simulink model "GNC_integrated_v3"  (R2023a)
settings: Solver=ode4  StartTime=0.0  StopTime=200  FixedStep=0.001  RelTol=1e-3
values from neighbouring files (symbols this model uses):
  baseMission = 1    [uavPackageDeliveryDataDict.sldd]
undefined symbols (not defined in the file or in its folder): Discrete, param, Time
libraries: dspfdesign x14, simulink_extras x6, uavalgslib x4, simulink x2, sharedTrackingLibrary x1, ctrlSharedLib x1, dspmtrx3 x1, SignalEditorBlockLib x1
settings Model: Creator=timme  LastModifiedBy=jipva

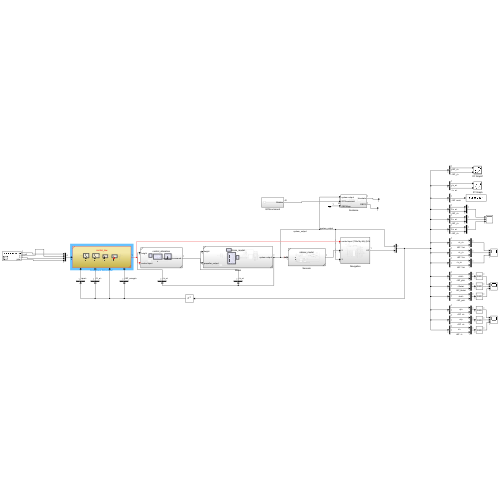
[thumbnail: Simulink's stored preview of the top-level diagram]
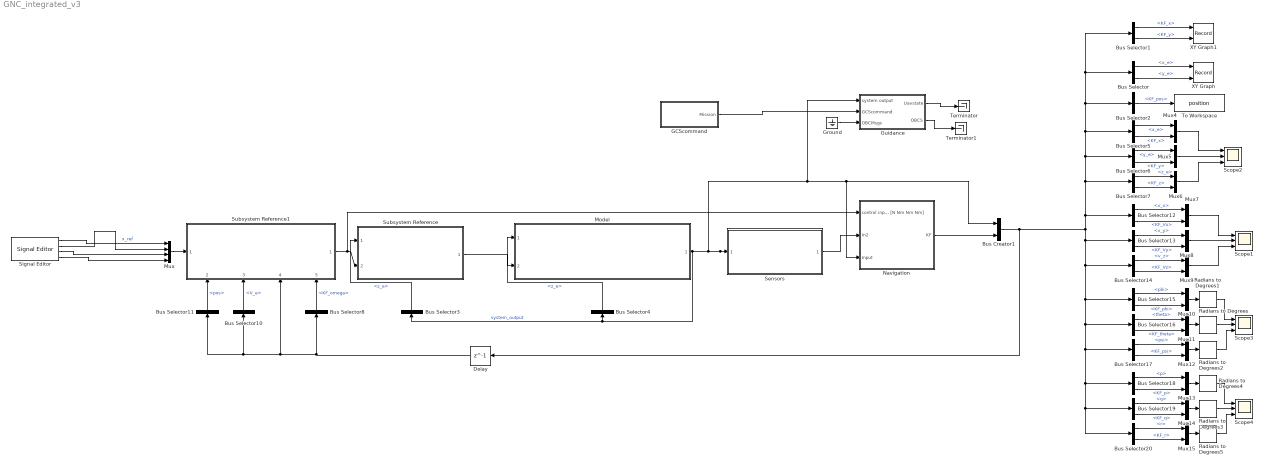
== system GNC_integrated_v3 ==
  Bus Creator1 : BusCreator  Inputs=2
  Bus Selector : BusSelector  OutputSignals=system_output.pos.x_e,system_output.pos.y_e
  Bus Selector1 : BusSelector  OutputSignals=KF.KF_pos.KF_x,KF.KF_pos.KF_y
  Bus Selector10 : BusSelector  OutputSignals=system_output.V_e
  Bus Selector11 : BusSelector  OutputSignals=system_output.pos
  Bus Selector12 : BusSelector  OutputSignals=system_output.V_e.v_x,KF.KF_vel.KF_Vx
  Bus Selector13 : BusSelector  OutputSignals=system_output.V_e.v_y,KF.KF_vel.KF_Vy
  Bus Selector14 : BusSelector  OutputSignals=system_output.V_e.v_z,KF.KF_vel.KF_Vz
  Bus Selector15 : BusSelector  OutputSignals=system_output.Att.phi,KF.KF_att.KF_phi
  Bus Selector16 : BusSelector  OutputSignals=system_output.Att.theta,KF.KF_att.KF_theta
  Bus Selector17 : BusSelector  OutputSignals=system_output.Att.psi,KF.KF_att.KF_psi
  Bus Selector18 : BusSelector  OutputSignals=system_output.ang_vel.p,KF.KF_omega.KF_p
  Bus Selector19 : BusSelector  OutputSignals=system_output.ang_vel.q,KF.KF_omega.KF_q
  Bus Selector2 : BusSelector  OutputSignals=KF.KF_pos
  Bus Selector20 : BusSelector  OutputSignals=system_output.ang_vel.r,KF.KF_omega.KF_r
  Bus Selector3 : BusSelector  OutputSignals=pos.z_e
  Bus Selector4 : BusSelector  OutputSignals=pos.z_e
  Bus Selector5 : BusSelector  OutputSignals=system_output.pos.x_e,KF.KF_pos.KF_x
  Bus Selector6 : BusSelector  OutputSignals=system_output.pos.y_e,KF.KF_pos.KF_y
  Bus Selector7 : BusSelector  OutputSignals=system_output.pos.z_e,KF.KF_pos.KF_z
  Bus Selector8 : BusSelector  OutputSignals=KF.KF_omega
  Delay : Delay  DelayLength=1
  GCScommand : Subsystem
  Ground : Ground
  Guidance : Subsystem
  Model : Subsystem  ReferencedSubsystem=drone_model
  Mux : Mux
  Mux{4..15} (12 alike) : Mux  Inputs=2
  Navigation : Subsystem
  Radians to Degrees{,1..5} (6 alike) : simulink_extras/Transformations/Radians to Degrees
  Scope{1..4} (4 alike) : Scope  NumInputPorts=3
  Sensors : Subsystem  ReferencedSubsystem=sensor_model
  Signal Editor : SignalEditorBlockLib/Signal Editor  FileName=full_system_reference.mat  ActiveScenario=StandardScenario  ActiveSignal=yaw  IsBus=off  OutputBusObjectStr=Bus: BusObject  SampleTime=param.dt  ZeroCross=off  OutputAfterFinalValue=Setting to zero  Unit=inherit  PreserveSignalName=on  ApplySigPropsToAllScenarios=on
  Subsystem Reference : Subsystem  ReferencedSubsystem=control_allocation
  Subsystem Reference1 : Subsystem  ReferencedSubsystem=control_law
      settings: PortSchema="{\"entries\":[{\"content\":{\"sides\":[{\"content\":{\"connectorIds\":[\"In1\"]},\"type\":\"ConnectorPlacement.EquallySpacedRectSide\",\"uuid\":\"cbb659e7-d19a-4e68-9ae7-e5e39426296b\"},{\"content\":{\"connectorIds\":[\"Out1\"],\"side\":\"RIGHT\"},\"type\":\"ConnectorPlacement.EquallySpacedRectSide\",\"uuid\":\"c9f08a4e-80d9-41bf-93e6-4cfd11b32426\"},{\"content\":{\"side\":\"TOP\"},\"type\":\"ConnectorPlacement.EquallySpacedRectSide\",\"uuid\":\"8eafc22d-128e-4ca7-9eba-2c3fd299252c\"},{\"content\":{\"connectorIds\":[\"In2\",\"In3\",\"In4\",\"In5\"],\"side\":\"BOTTOM\"},\"type\":\"ConnectorPlacement.EquallySpacedRectSide\",\"uuid\":\"abe1dc09-e6b8-433e-beaf-ba54ebcb4b47\"}]},\"type\":\"ConnectorPlacement.EquallySpacedConnector\",\"uuid\":\"085ffc95-65e8-4235-be8d-72c324b16b8b\"}],\"packageUris\":[\"http://schema.mathworks.com/mf0/Connector/R2020b\"],\"version\":\"1.0\"}"
  Terminator : Terminator
  Terminator1 : Terminator
  To Workspace : ToWorkspace  VariableName=position  SaveFormat=Timeseries  SampleTime=0.001
  XY Graph : Record  FileSettingsInternal="{\"entries\":[{\"content\":{\"excelSettings\":{\"content\":{},\"type\":\"Streamout.ExcelSettings\"}},\"type\":\"Streamout.FileSettingStorage\",\"uuid\":\"\"}],\"packageUris\":[\"http:\\/\\/schema.mathworks.com\\/mf0\\/streamout_blocks\\/R2020a\"],\"version\":\"1.0\"}"  Layout=[1 1]  SignalsInternal="{\"entries\":[{\"content\":{\"signals\":[{\"content\":{\"blockPath\":[],\"dimensions\":[1],\"domain\":\"\",\"lineColor\":\"#a2142f\",\"plots\":[1],\"port\":1,\"signalID\":16,\"signalName\":\"<x_e>\"},\"type\":\"RecordBlkView.Signal\",\"uuid\":\"\"},{\"content\":{\"blockPath\":[],\"dimensions\":[1],\"domain\":\"\",\"lineColor\":\"#139fff\",\"plots\":[1],\"port\":2,\"signalID\":19,\"signalName\":\"<y_e>\"},\"type\":\"RecordBlkView.Signal\",\"uuid\":\"\"}]},\"type\":\"RecordBlkView.InputSignals\",\"uuid\":\"\"}],\"packageUris\":[\"http:\\/\\/schema.mathworks.com\\/mf0\\/streamout_blocks\\/R2020a\"],\"version\":\"1.0\"}"  VisualizationBindings="{\"xyplotplugin\":{\"info\":[{\"series\":[{\"bindingParametersList\":[{\"parameter\":\"X-Axis\",\"signalID\":16,\"signalName\":\"<x_e>\"},{\"parameter\":\"Y-Axis\",\"signalID\":19,\"signalName\":\"<y_e>\"}],\"seriesID\":45778}],\"subplotID\":1}]}}"  CompatibilityTag=XY
  XY Graph1 : Record  FileSettingsInternal="{\"entries\":[{\"content\":{\"excelSettings\":{\"content\":{},\"type\":\"Streamout.ExcelSettings\"}},\"type\":\"Streamout.FileSettingStorage\",\"uuid\":\"\"}],\"packageUris\":[\"http:\\/\\/schema.mathworks.com\\/mf0\\/streamout_blocks\\/R2020a\"],\"version\":\"1.0\"}"  Layout=[1 1]  SignalsInternal="{\"entries\":[{\"content\":{\"signals\":[{\"content\":{\"blockPath\":[],\"dimensions\":[1,1],\"domain\":\"\",\"lineColor\":\"#a2142f\",\"plots\":[1],\"port\":1,\"signalID\":8,\"signalName\":\"<KF_x>\"},\"type\":\"RecordBlkView.Signal\",\"uuid\":\"\"},{\"content\":{\"blockPath\":[],\"dimensions\":[1,1],\"domain\":\"\",\"lineColor\":\"#139fff\",\"plots\":[1],\"port\":2,\"signalID\":11,\"signalName\":\"<KF_y>\"},\"type\":\"RecordBlkView.Signal\",\"uuid\":\"\"}]},\"type\":\"RecordBlkView.InputSignals\",\"uuid\":\"\"}],\"packageUris\":[\"http:\\/\\/schema.mathworks.com\\/mf0\\/streamout_blocks\\/R2020a\"],\"version\":\"1.0\"}"  VisualizationBindings="{\"xyplotplugin\":{\"info\":[{\"series\":[{\"bindingParametersList\":[{\"parameter\":\"X-Axis\",\"signalID\":8,\"signalName\":\"<KF_x>\"},{\"parameter\":\"Y-Axis\",\"signalID\":11,\"signalName\":\"<KF_y>\"}],\"seriesID\":47810}],\"subplotID\":1}]}}"  CompatibilityTag=XY
  wires:
  Bus Selector5/1 -> Mux4/1  "<x_e>"
  Bus Selector5/2 -> Mux4/2  "<KF_x>"
  Bus Selector6/1 -> Mux5/1  "<y_e>"
  Bus Selector6/2 -> Mux5/2  "<KF_y>"
  Bus Selector7/2 -> Mux6/2  "<KF_z>"
  Bus Selector7/1 -> Mux6/1  "<z_e>"
  Bus Selector12/2 -> Mux7/2  "<KF_Vx>"
  Bus Selector12/1 -> Mux7/1  "<v_x>"
  Bus Selector13/1 -> Mux8/1  "<v_y>"
  Bus Selector14/2 -> Mux9/2  "<KF_Vz>"
  Bus Selector14/1 -> Mux9/1  "<v_z>"
  Bus Selector13/2 -> Mux8/2  "<KF_Vy>"
  Bus Selector16/2 -> Mux11/2  "<KF_theta>"
  Mux12/1 -> Radians to Degrees2/1
  Mux11/1 -> Radians to Degrees/1
  Bus Selector17/2 -> Mux12/2  "<KF_psi>"
  Bus Selector17/1 -> Mux12/1  "<psi>"
  Bus Selector15/2 -> Mux10/2  "<KF_phi>"
  Mux10/1 -> Radians to Degrees1/1
  Bus Selector15/1 -> Mux10/1  "<phi>"
  Bus Selector16/1 -> Mux11/1  "<theta>"
  Bus Selector19/2 -> Mux14/2  "<KF_q>"
  Bus Selector18/2 -> Mux13/2  "<KF_p>"
  Mux13/1 -> Radians to Degrees4/1
  Bus Selector20/1 -> Mux15/1  "<r>"
  Bus Selector18/1 -> Mux13/1  "<p>"
  Mux15/1 -> Radians to Degrees5/1
  Bus Selector20/2 -> Mux15/2  "<KF_r>"
  Mux14/1 -> Radians to Degrees3/1
  Bus Selector19/1 -> Mux14/1  "<q>"
  Signal Editor/1 -> Mux/1  "x_ref"
  Bus Selector/1 -> XY Graph/1  "<x_e>"
  Bus Selector/2 -> XY Graph/2  "<y_e>"
  Mux5/1 -> Scope2/2
  Mux4/1 -> Scope2/1
  Mux6/1 -> Scope2/3
  Mux8/1 -> Scope1/2
  Mux9/1 -> Scope1/3
  Mux7/1 -> Scope1/1
  Radians to Degrees2/1 -> Scope3/3
  Radians to Degrees1/1 -> Scope3/1
  Radians to Degrees/1 -> Scope3/2
  Radians to Degrees5/1 -> Scope4/3
  Radians to Degrees4/1 -> Scope4/1
  Radians to Degrees3/1 -> Scope4/2
  Bus Selector1/1 -> XY Graph1/1  "<KF_x>"
  Bus Selector1/2 -> XY Graph1/2  "<KF_y>"
  Sensors/1 -> Navigation/2(In2)
  Navigation/1(KF) -> Bus Creator1/2
  Bus Selector2/1 -> To Workspace/1  "<KF_pos>"
  Bus Creator1/1 -> Delay/1, Bus Selector13/1, Bus Selector14/1, Bus Selector20/1, Bus Selector19/1, Bus Selector18/1, Bus Selector17/1, Bus Selector16/1, Bus Selector15/1, Bus Selector12/1, Bus Selector7/1, Bus Selector6/1, Bus Selector2/1, Bus Selector1/1, Bus Selector/1, Bus Selector5/1
  Mux/1 -> Subsystem Reference1/1
  Bus Selector11/1 -> Subsystem Reference1/2  "<pos>"
  Bus Selector10/1 -> Subsystem Reference1/3  "<V_e>"
  Delay/1 -> Bus Selector8/1, Subsystem Reference1/4, Bus Selector11/1, Bus Selector10/1
  Bus Selector8/1 -> Subsystem Reference1/5  "<KF_omega>"
  Bus Selector3/1 -> Subsystem Reference/1  "<z_e>"
  Bus Selector4/1 -> Model/1  "<z_e>"
  Signal Editor/4 -> Mux/4
  Signal Editor/3 -> Mux/3
  Signal Editor/2 -> Mux/2
  Subsystem Reference1/1 -> Subsystem Reference/2, Navigation/1(control input (T Mx My Mz) [N Nm Nm Nm])
  Subsystem Reference/1 -> Model/2
  Model/1 -> Bus Selector3/1, Bus Selector4/1, Sensors/1, Guidance/1(system output), Navigation/3(Input), Bus Creator1/1  "system_output"
  Guidance/2(OBCS) -> Terminator1/1
  Ground/1 -> Guidance/3(OBCMsgs)
  Guidance/1(Uavstate) -> Terminator/1
  GCScommand/1(Mission) -> Guidance/2(GCScommand)

== system GNC_integrated_v3/GCScommand ==
  Constant : Constant  Value=baseMission  OutDataTypeStr=Bus: UAVPathManagerBus  SampleTime=-1
  Mission : Outport
  wires:
  Constant/1 -> Mission/1

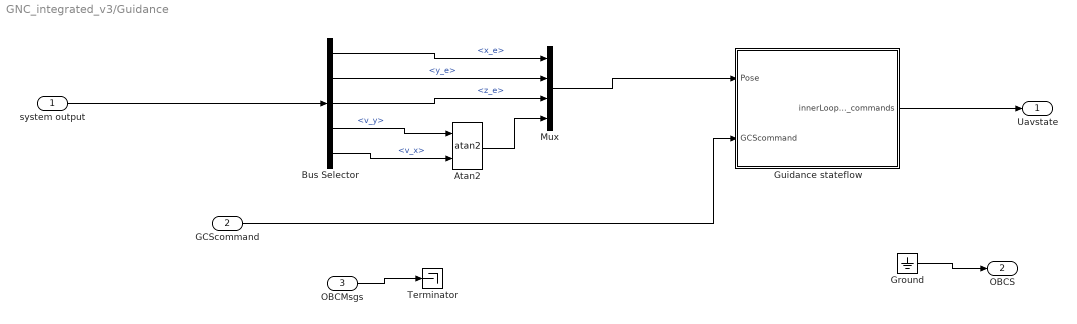
== system GNC_integrated_v3/Guidance ==
  system output : Inport
  GCScommand : Inport  Port=2
  OBCMsgs : Inport  Port=3
  Atan2 : Trigonometry  Operator=atan2
  Bus Selector : BusSelector  OutputSignals=pos.x_e,pos.y_e,pos.z_e,V_e.v_y,V_e.v_x
  Ground : Ground
  Guidance stateflow : Subsystem
  Mux : Mux
  Terminator : Terminator
  Uavstate : Outport
  OBCS : Outport  Port=2
  wires:
  Bus Selector/4 -> Atan2/1  "<v_y>"
  Bus Selector/5 -> Atan2/2  "<v_x>"
  Bus Selector/3 -> Mux/3  "<z_e>"
  Bus Selector/2 -> Mux/2  "<y_e>"
  Bus Selector/1 -> Mux/1  "<x_e>"
  Atan2/1 -> Mux/4
  Mux/1 -> Guidance stateflow/1(Pose)
  GCScommand/1 -> Guidance stateflow/2(GCScommand)
  OBCMsgs/1 -> Terminator/1
  Guidance stateflow/1(innerLoop_commands) -> Uavstate/1
  Ground/1 -> OBCS/1
  system output/1 -> Bus Selector/1

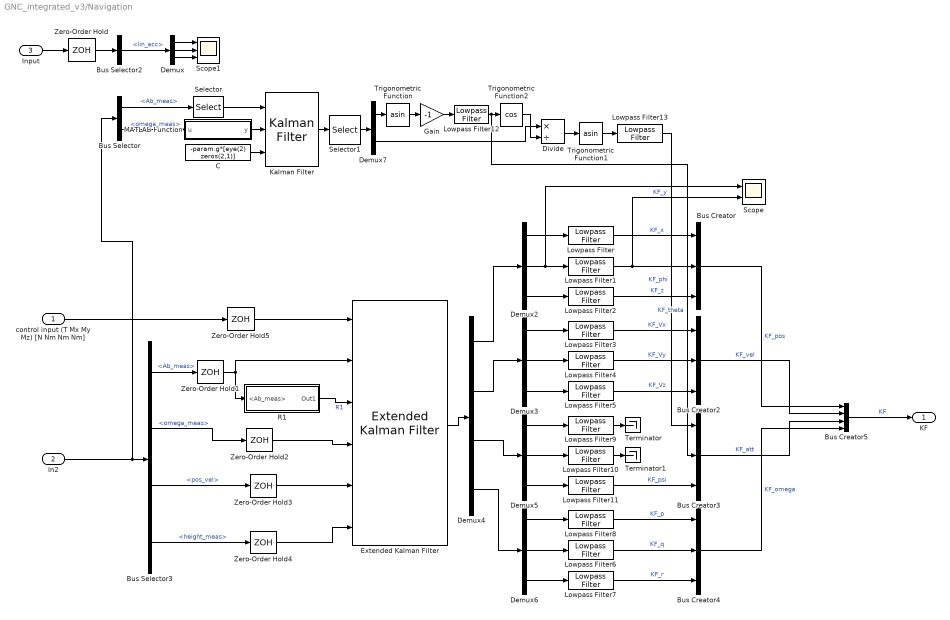
== system GNC_integrated_v3/Navigation ==
  control input (T Mx My Mz) [N Nm Nm Nm] : Inport
  In2 : Inport  Port=2
  Input : Inport  Port=3
  Bus Creator{,2..4} (4 alike) : BusCreator  Inputs=3
  Bus Creator5 : BusCreator  Inputs=4
  Bus Selector : BusSelector  OutputSignals=Ab_meas,omega_meas
  Bus Selector2 : BusSelector  OutputSignals=lin_acc
  Bus Selector3 : BusSelector  OutputSignals=Ab_meas,omega_meas,pos_vel,height_meas
  C : Constant  Value=-param.g*[eye(2) zeros(2,1)]
  Demux{,2..3,5..6} (5 alike) : Demux  Outputs=3
  Demux4 : Demux
  Demux7 : Demux  Outputs=2
  Divide : Product  Inputs=*/
  Extended Kalman Filter : sharedTrackingLibrary/Extended Kalman Filter  StateTransitionFcn=stateTransition  HasStateTransitionJacobianFcn=off  HasAdditiveProcessNoise=Additive  ProcessNoise=diag([1*ones(1,6) [1 1 0.01] [0.1 0.1 0.1]])  HasTimeVaryingProcessNoise=off  HasStateTransitionFcnExtraArgument=1  InitialState=zeros(12,1)  InitialStateCovariance=zeros(12)  MeasurementFcn1=accelerometer_model  HasMeasurementJacobianFcn1=off  HasMeasurementEnablePort1=off  HasAdditiveMeasurementNoise1=Additive  MeasurementNoise1=diag([20 20 20])  HasTimeVaryingMeasurementNoise1=on  HasMeasurementFcnExtraArgument1=0  HasMeasurementWrapping1=off  MeasurementFcn2=gyrometer_model  HasMeasurementJacobianFcn2=off  HasMeasurementEnablePort2=off  HasAdditiveMeasurementNoise2=Additive  MeasurementNoise2=diag([1 1 10])  HasTimeVaryingMeasurementNoise2=off  HasMeasurementFcnExtraArgument2=0  HasMeasurementWrapping2=off  MeasurementFcn3=GPS_model  HasMeasurementJacobianFcn3=off  HasMeasurementEnablePort3=off  HasAdditiveMeasurementNoise3=Additive  MeasurementNoise3=diag([0.001 0.001 0.001 0.001 0.001 0.001])  HasTimeVaryingMeasurementNoise3=off  HasMeasurementFcnExtraArgument3=0  HasMeasurementWrapping3=off  MeasurementFcn4=Barometer_model  HasMeasurementJacobianFcn4=off  HasMeasurementEnablePort4=off  HasAdditiveMeasurementNoise4=Additive  MeasurementNoise4=0.01  HasTimeVaryingMeasurementNoise4=off  HasMeasurementFcnExtraArgument4=0  HasMeasurementWrapping4=off  MeasurementFcn5=myMeasurementFcn  HasMeasurementJacobianFcn5=off  HasMeasurementEnablePort5=off  HasAdditiveMeasurementNoise5=Additive  MeasurementNoise5=1  HasTimeVaryingMeasurementNoise5=off  HasMeasurementFcnExtraArgument5=0  HasMeasurementWrapping5=off  EnableMultirate=on  StateTransitionFcnSampleTime=0.001  MeasurementFcn1SampleTime=0.001  MeasurementFcn2SampleTime=0.001  MeasurementFcn3SampleTime=0.001  MeasurementFcn4SampleTime=0.01  MeasurementFcn5SampleTime=1  UseCurrentEstimator=on  OutputStateCovariance=off  DataType=double  SampleTime=0.001  NumberOfMeasurements=4
  Gain : Gain  Gain=-1
  Kalman Filter : ctrlSharedLib/Kalman Filter  TimeDomain=Discrete-Time  UseCurrentEstimator=on  ModelSource=Input port  ModelSourceVariable=ss(0.95,1,1,0,1)  A=0.95  B=1  C=1  D=0  NumberOfStates=3  NumberOfInputs=1  NumberOfOutputs=2  InitialEstimateSource=Dialog  X0=0  P0=1  UseK=off  UseGH=off  NumberOfProcessNoiseInputs=1  G=eye(3)  TimeInvariantG=on  H=ones(2,1)  TimeInvariantH=on  Q=100  TimeInvariantQ=on  R=0.0001  TimeInvariantR=on  N=0  TimeInvariantN=on  AddInputPort=off  AddEnablePort=off  OutputEstimatedY=off  OutputP=off  Ts=0.001
  Lowpass Filter : dspfdesign/Lowpass Filter  FilterType=IIR  DesignForMinimumOrder=on  FilterOrder=50  PassbandFrequency=1  StopbandFrequency=499  PassbandRipple=0.1  StopbandAttenuation=80  SampleRateMode=Specify on dialog  SampleRate=1000  SimulateUsing=Interpreted execution  roundingMode=Floor  coeffsDataTypeStr=fixdt(1,16)
  Lowpass Filter1 : dspfdesign/Lowpass Filter  FilterType=IIR  DesignForMinimumOrder=on  FilterOrder=50  PassbandFrequency=1  StopbandFrequency=499  PassbandRipple=0.1  StopbandAttenuation=80  SampleRateMode=Specify on dialog  SampleRate=1000  SimulateUsing=Interpreted execution  roundingMode=Floor  coeffsDataTypeStr=fixdt(1,16)
  Lowpass Filter10 : dspfdesign/Lowpass Filter  FilterType=IIR  DesignForMinimumOrder=on  FilterOrder=50  PassbandFrequency=0.1  StopbandFrequency=25  PassbandRipple=0.1  StopbandAttenuation=80  SampleRateMode=Specify on dialog  SampleRate=1000  SimulateUsing=Interpreted execution  roundingMode=Floor  coeffsDataTypeStr=fixdt(1,16)
  Lowpass Filter11 : dspfdesign/Lowpass Filter  FilterType=IIR  DesignForMinimumOrder=on  FilterOrder=50  PassbandFrequency=0.1  StopbandFrequency=25  PassbandRipple=0.1  StopbandAttenuation=80  SampleRateMode=Specify on dialog  SampleRate=1000  SimulateUsing=Interpreted execution  roundingMode=Floor  coeffsDataTypeStr=fixdt(1,16)
  Lowpass Filter{6..8,12..13} (5 alike) : dspfdesign/Lowpass Filter  FilterType=IIR  DesignForMinimumOrder=on  FilterOrder=50  PassbandFrequency=5  StopbandFrequency=60  PassbandRipple=0.1  StopbandAttenuation=45  SampleRateMode=Specify on dialog  SampleRate=1000  SimulateUsing=Interpreted execution  roundingMode=Floor  coeffsDataTypeStr=fixdt(1,16)
  Lowpass Filter2 : dspfdesign/Lowpass Filter  FilterType=IIR  DesignForMinimumOrder=on  FilterOrder=50  PassbandFrequency=1  StopbandFrequency=499  PassbandRipple=0.1  StopbandAttenuation=80  SampleRateMode=Specify on dialog  SampleRate=1000  SimulateUsing=Interpreted execution  roundingMode=Floor  coeffsDataTypeStr=fixdt(1,16)
  Lowpass Filter3 : dspfdesign/Lowpass Filter  FilterType=IIR  DesignForMinimumOrder=on  FilterOrder=50  PassbandFrequency=0.1  StopbandFrequency=10  PassbandRipple=0.1  StopbandAttenuation=80  SampleRateMode=Specify on dialog  SampleRate=1000  SimulateUsing=Interpreted execution  roundingMode=Floor  coeffsDataTypeStr=fixdt(1,16)
  Lowpass Filter4 : dspfdesign/Lowpass Filter  FilterType=IIR  DesignForMinimumOrder=on  FilterOrder=50  PassbandFrequency=0.1  StopbandFrequency=50  PassbandRipple=0.1  StopbandAttenuation=80  SampleRateMode=Specify on dialog  SampleRate=1000  SimulateUsing=Interpreted execution  roundingMode=Floor  coeffsDataTypeStr=fixdt(1,16)
  Lowpass Filter5 : dspfdesign/Lowpass Filter  FilterType=IIR  DesignForMinimumOrder=on  FilterOrder=50  PassbandFrequency=0.1  StopbandFrequency=50  PassbandRipple=0.1  StopbandAttenuation=80  SampleRateMode=Specify on dialog  SampleRate=1000  SimulateUsing=Interpreted execution  roundingMode=Floor  coeffsDataTypeStr=fixdt(1,16)
  Lowpass Filter9 : dspfdesign/Lowpass Filter  FilterType=IIR  DesignForMinimumOrder=on  FilterOrder=50  PassbandFrequency=0.1  StopbandFrequency=25  PassbandRipple=0.1  StopbandAttenuation=80  SampleRateMode=Specify on dialog  SampleRate=1000  SimulateUsing=Interpreted execution  roundingMode=Floor  coeffsDataTypeStr=fixdt(1,16)
  MATLAB Function : MATLAB Function  TreatAsAtomicUnit=on
  R1 : Subsystem
  Scope : Scope  NumInputPorts=2
  Scope1 : Scope  NumInputPorts=3
  Selector : Selector  InputPortWidth=3  IndexOptions=Index vector (dialog)  Indices=[1 2]  OutputSizes=1
  Selector1 : Selector  InputPortWidth=3  IndexOptions=Index vector (dialog)  Indices=[1 2]  OutputSizes=1
  Terminator : Terminator
  Terminator1 : Terminator
  Trigonometric Function : Trigonometry  Operator=asin
  Trigonometric Function1 : Trigonometry  Operator=asin
  Trigonometric Function2 : Trigonometry  Operator=cos
  Zero-Order Hold{,1..3,5} (5 alike) : ZeroOrderHold  SampleTime=0.001
  Zero-Order Hold4 : ZeroOrderHold  SampleTime=0.01
  KF : Outport
  wires:
  Demux5/2 -> Lowpass Filter10/1
  Bus Selector3/2 -> Zero-Order Hold2/1  "<omega_meas>"
  Bus Selector3/3 -> Zero-Order Hold3/1  "<pos_vel>"
  Demux2/3 -> Lowpass Filter2/1
  Zero-Order Hold5/1 -> Extended Kalman Filter/1
  Demux3/1 -> Lowpass Filter3/1
  In2/1 -> Bus Selector3/1, Bus Selector/1
  Demux5/3 -> Lowpass Filter11/1
  Bus Creator2/1 -> Bus Creator5/2  "KF_vel"
  Bus Creator/1 -> Bus Creator5/1  "KF_pos"
  Demux4/2 -> Demux3/1
  Demux3/3 -> Lowpass Filter5/1
  Demux2/1 -> Lowpass Filter/1
  Demux4/1 -> Demux2/1
  Demux5/1 -> Lowpass Filter9/1
  Zero-Order Hold1/1 -> Extended Kalman Filter/2, R1/1(<Ab_meas>)
  Demux3/2 -> Lowpass Filter4/1
  Bus Selector3/4 -> Zero-Order Hold4/1  "<height_meas>"
  Bus Creator3/1 -> Bus Creator5/3  "KF_att"
  Demux4/4 -> Demux6/1
  Lowpass Filter1/1 -> Scope/2, Bus Creator/2  "KF_y"
  Extended Kalman Filter/1 -> Demux4/1
  Demux4/3 -> Demux5/1
  Bus Creator5/1 -> KF/1  "KF"
  control input (T Mx My Mz) [N Nm Nm Nm]/1 -> Zero-Order Hold5/1
  Lowpass Filter/1 -> Bus Creator/1  "KF_x"
  Demux2/2 -> Scope/1, Lowpass Filter1/1
  Lowpass Filter2/1 -> Bus Creator/3  "KF_z"
  Lowpass Filter3/1 -> Bus Creator2/1  "KF_Vx"
  Lowpass Filter4/1 -> Bus Creator2/2  "KF_Vy"
  Lowpass Filter5/1 -> Bus Creator2/3  "KF_Vz"
  Lowpass Filter11/1 -> Bus Creator3/3  "KF_psi"
  Lowpass Filter8/1 -> Bus Creator4/1  "KF_p"
  Lowpass Filter6/1 -> Bus Creator4/2  "KF_q"
  Lowpass Filter7/1 -> Bus Creator4/3  "KF_r"
  Demux6/1 -> Lowpass Filter8/1
  Demux6/2 -> Lowpass Filter6/1
  Demux6/3 -> Lowpass Filter7/1
  Zero-Order Hold2/1 -> Extended Kalman Filter/4
  Zero-Order Hold3/1 -> Extended Kalman Filter/5
  Zero-Order Hold4/1 -> Extended Kalman Filter/6
  R1/1(Out1) -> Extended Kalman Filter/3  "R1"
  Bus Selector3/1 -> Zero-Order Hold1/1  "<Ab_meas>"
  Bus Creator4/1 -> Bus Creator5/4  "KF_omega"
  Bus Selector/1 -> Selector/1  "<Ab_meas>"
  C/1 -> Kalman Filter/3
  Bus Selector/2 -> MATLAB Function/1(u)  "<omega_meas>"
  MATLAB Function/1(y) -> Kalman Filter/2
  Kalman Filter/1 -> Selector1/1
  Demux7/1 -> Trigonometric Function/1
  Selector/1 -> Kalman Filter/1
  Gain/1 -> Lowpass Filter12/1
  Trigonometric Function/1 -> Gain/1
  Demux7/2 -> Divide/1
  Lowpass Filter12/1 -> Bus Creator3/2, Trigonometric Function2/1  "KF_theta"
  Input/1 -> Zero-Order Hold/1
  Zero-Order Hold/1 -> Bus Selector2/1
  Lowpass Filter13/1 -> Bus Creator3/1  "KF_phi"
  Divide/1 -> Trigonometric Function1/1
  Selector1/1 -> Demux7/1
  Trigonometric Function1/1 -> Lowpass Filter13/1
  Trigonometric Function2/1 -> Divide/2
  Lowpass Filter9/1 -> Terminator/1
  Lowpass Filter10/1 -> Terminator1/1
  Bus Selector2/1 -> Demux/1  "<lin_acc>"
  Demux/2 -> Scope1/2
  Demux/1 -> Scope1/1
  Demux/3 -> Scope1/3

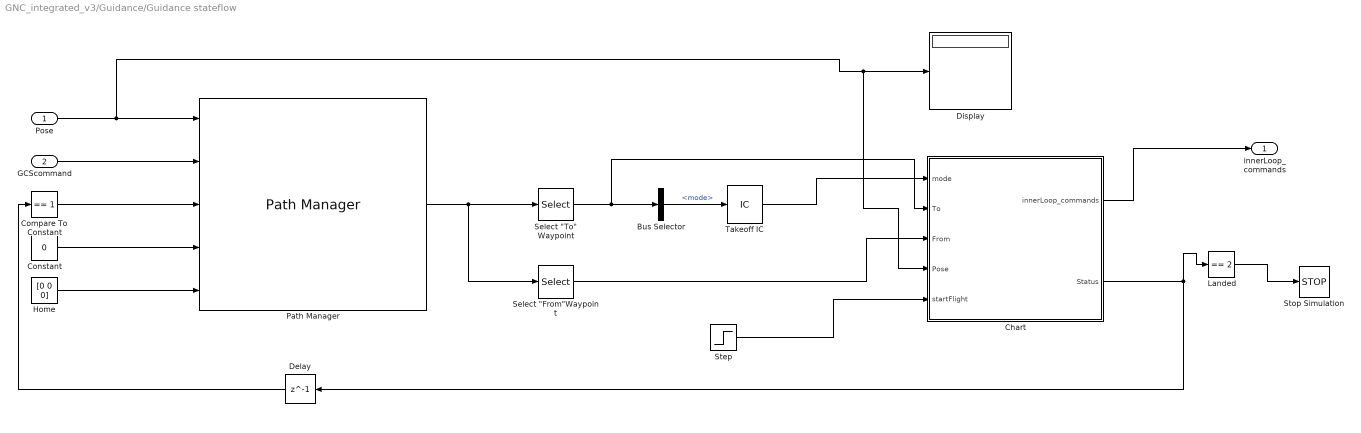
== system GNC_integrated_v3/Guidance/Guidance stateflow ==
  Pose : Inport
  GCScommand : Inport  Port=2
  Bus Selector : BusSelector  OutputSignals=mode
  Chart : Stateflow chart  TreatAsAtomicUnit=on
  Compare To Constant : simulink/Logic and Bit Operations/Compare To Constant  relop===  const=1  OutDataTypeStr=boolean
  Constant : Constant  Value=0  OutDataTypeStr=uint8
  Delay : Delay  DelayLength=1  InitialCondition=0
  Display : Display
  Home : Constant  Value=[0 0 0]
  Landed : simulink/Logic and Bit Operations/Compare To Constant  relop===  const=2  OutDataTypeStr=boolean
  Path Manager : uavalgslib/Path Manager  UAVType=multirotor  LoiterRadius=25  dataType=single  inputBusName='UAVPathManagerBus'  SimulateUsing=Code generation
  "Select \"From\"Waypoint" : Selector  InputPortWidth=2  IndexOptions=Index vector (dialog)  Indices=2  OutputSizes=1
  "Select \"To\" Waypoint" : Selector  InputPortWidth=2  IndexOptions=Index vector (dialog)  Indices=1  OutputSizes=1
  Step : Step  Time=0.5  SampleTime=0.02
  Stop Simulation : Stop
  Takeoff IC : InitialCondition
  innerLoop_commands : Outport
  wires:
  GCScommand/1 -> Path Manager/2
  Home/1 -> Path Manager/5
  Constant/1 -> Path Manager/4
  Path Manager/1 -> "Select \"From\"Waypoint"/1, "Select \"To\" Waypoint"/1
  Bus Selector/1 -> Takeoff IC/1  "<mode>"
  Delay/1 -> Compare To Constant/1
  Compare To Constant/1 -> Path Manager/3
  Step/1 -> Chart/5(startFlight)
  Landed/1 -> Stop Simulation/1
  Pose/1 -> Chart/4(Pose), Display/1, Path Manager/1
  "Select \"To\" Waypoint"/1 -> Chart/2(To), Bus Selector/1
  "Select \"From\"Waypoint"/1 -> Chart/3(From)
  Takeoff IC/1 -> Chart/1(mode)
  Chart/1(innerLoop_commands) -> innerLoop_commands/1
  Chart/2(Status) -> Landed/1, Delay/1

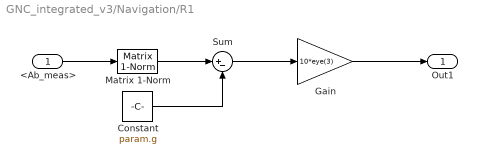
== system GNC_integrated_v3/Navigation/R1 ==
  <Ab_meas> : Inport
  Constant : Constant  Value=param.g
  Gain : Gain  Gain=10*eye(3)
  Matrix 1-Norm : dspmtrx3/Matrix  1-Norm  roundingMode=Floor  overflowMode=off  outputDataTypeStr=Inherit: Same as accumulator  outputMin=[]  outputMax=[]  outputLastDataTypeStr=Inherit: Same as accumulator
  Sum : Sum  Inputs=|+-
  Out1 : Outport
  wires:
  Matrix 1-Norm/1 -> Sum/1
  <Ab_meas>/1 -> Matrix 1-Norm/1
  Constant/1 -> Sum/2
  Sum/1 -> Gain/1
  Gain/1 -> Out1/1

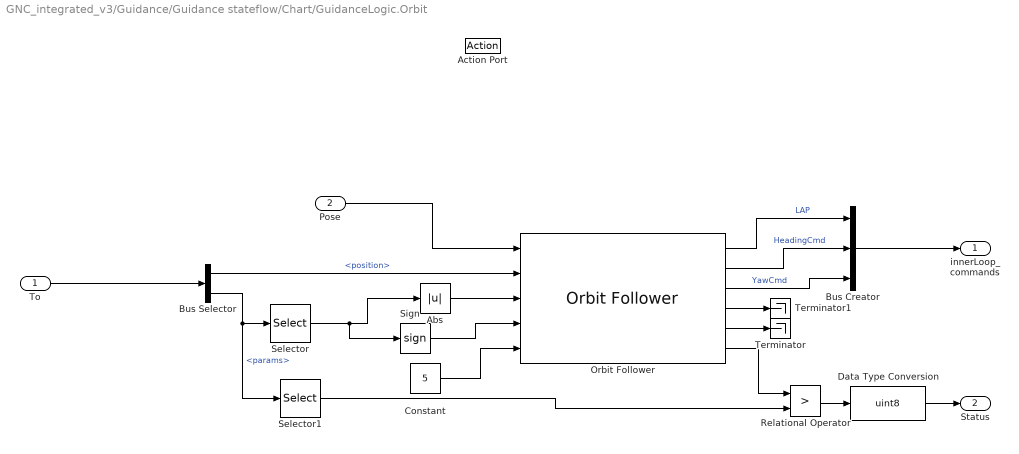
== system GNC_integrated_v3/Guidance/Guidance stateflow/Chart/GuidanceLogic.Orbit ==
  To : Inport
  Pose : Inport  Port=2
  Action Port : ActionPort
      settings: CopyFcn=Stateflow.SLINSF.SimulinkMan.removeBlockPreDeleteFcn  PreDeleteFcn=Stateflow.SLINSF.SimulinkMan.unsafePredeleteFcn
  Abs : Abs  SaturateOnIntegerOverflow=off
  Bus Creator : BusCreator  Inputs=3  OutDataTypeStr=Bus: innerLoopCmdsBus  NonVirtualBus=on
  Bus Selector : BusSelector  OutputSignals=position,params
  Constant : Constant  Value=5  OutDataTypeStr=uint8
  Data Type Conversion : DataTypeConversion  OutDataTypeStr=uint8  SaturateOnIntegerOverflow=off  RndMeth=Floor
  Orbit Follower : uavalgslib/Orbit Follower  UAVType=multirotor  MinOrbitRadius=1  MinLookaheadDistance=0.1  ExternalReset=none  ShowCrossTrackErrorOutput=off  ShowNumTurnsOutput=on  SimulateUsing=Code generation
  Relational Operator : RelationalOperator  Operator=>  OutDataTypeStr=boolean  RndMeth=Simplest  InputSameDT=off
  Selector : Selector  InputPortWidth=4  IndexOptions=Index vector (dialog)  Indices=[3]  OutputSizes=1
  Selector1 : Selector  InputPortWidth=4  IndexOptions=Index vector (dialog)  Indices=[1]  OutputSizes=1
  Sign : Signum
  Terminator : Terminator
  Terminator1 : Terminator
  innerLoop_commands : Outport
  Status : Outport  Port=2
  wires:
  To/1 -> Bus Selector/1
  Orbit Follower/4 -> Terminator1/1
  Orbit Follower/5 -> Terminator/1
  Orbit Follower/1 -> Bus Creator/1  "LAP"
  Orbit Follower/2 -> Bus Creator/2  "HeadingCmd"
  Orbit Follower/3 -> Bus Creator/3  "YawCmd"
  Bus Creator/1 -> innerLoop_commands/1
  Pose/1 -> Orbit Follower/1
  Bus Selector/1 -> Orbit Follower/2  "<position>"
  Bus Selector/2 -> Selector1/1, Selector/1  "<params>"
  Abs/1 -> Orbit Follower/3
  Selector/1 -> Sign/1, Abs/1
  Constant/1 -> Orbit Follower/5
  Sign/1 -> Orbit Follower/4
  Orbit Follower/6 -> Relational Operator/1
  Selector1/1 -> Relational Operator/2
  Relational Operator/1 -> Data Type Conversion/1
  Data Type Conversion/1 -> Status/1

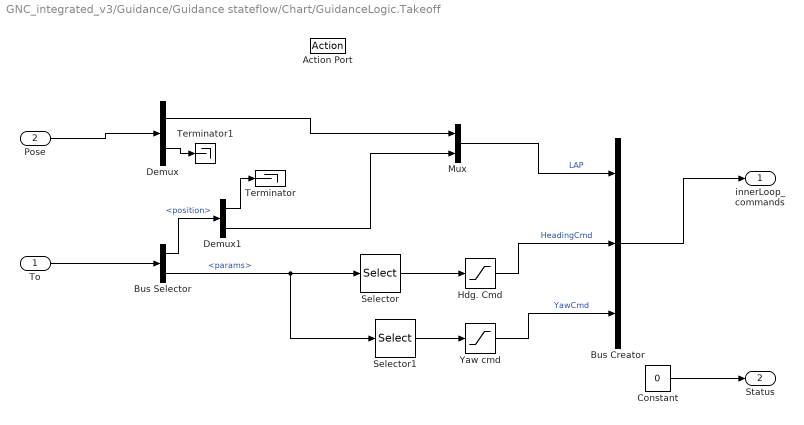
== system GNC_integrated_v3/Guidance/Guidance stateflow/Chart/GuidanceLogic.Takeoff ==
  To : Inport
  Pose : Inport  Port=2
  Action Port : ActionPort
      settings: CopyFcn=Stateflow.SLINSF.SimulinkMan.removeBlockPreDeleteFcn  PreDeleteFcn=Stateflow.SLINSF.SimulinkMan.unsafePredeleteFcn
  Bus Creator : BusCreator  Inputs=3  OutDataTypeStr=Bus: innerLoopCmdsBus  NonVirtualBus=on
  Bus Selector : BusSelector  OutputSignals=position,params
  Constant : Constant  Value=0
  Demux : Demux  Outputs=[2 2]
  Demux1 : Demux  Outputs=2
  Hdg. Cmd : Saturate
  Mux : Mux  Inputs=2
  Selector : Selector  InputPortWidth=4  IndexOptions=Index vector (dialog)  Indices=4  OutputSizes=1
  Selector1 : Selector  InputPortWidth=4  IndexOptions=Index vector (dialog)  Indices=4  OutputSizes=1
  Terminator : Terminator
  Terminator1 : Terminator
  Yaw cmd : Saturate  UpperLimit=pi  LowerLimit=-pi
  innerLoop_commands : Outport
  Status : Outport  Port=2  OutDataTypeStr=uint8
  wires:
  Pose/1 -> Demux/1
  Demux/1 -> Mux/1
  Mux/1 -> Bus Creator/1  "LAP"
  To/1 -> Bus Selector/1
  Bus Selector/1 -> Demux1/1  "<position>"
  Demux1/1 -> Terminator/1
  Demux1/2 -> Mux/2
  Bus Selector/2 -> Selector1/1, Selector/1  "<params>"
  Bus Creator/1 -> innerLoop_commands/1
  Demux/2 -> Terminator1/1
  Hdg. Cmd/1 -> Bus Creator/2  "HeadingCmd"
  Selector1/1 -> Yaw cmd/1
  Selector/1 -> Hdg. Cmd/1
  Yaw cmd/1 -> Bus Creator/3  "YawCmd"
  Constant/1 -> Status/1

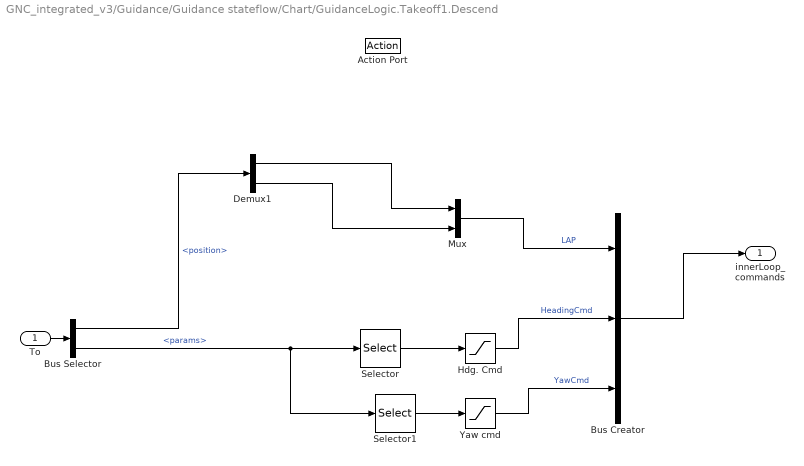
== system GNC_integrated_v3/Guidance/Guidance stateflow/Chart/GuidanceLogic.Takeoff1.Descend ==
  To : Inport
  Action Port : ActionPort
      settings: CopyFcn=Stateflow.SLINSF.SimulinkMan.removeBlockPreDeleteFcn  PreDeleteFcn=Stateflow.SLINSF.SimulinkMan.unsafePredeleteFcn
  Bus Creator : BusCreator  Inputs=3  OutDataTypeStr=Bus: innerLoopCmdsBus  NonVirtualBus=on
  Bus Selector : BusSelector  OutputSignals=position,params
  Demux1 : Demux  Outputs=[2 1]
  Hdg. Cmd : Saturate
  Mux : Mux  Inputs=2
  Selector : Selector  InputPortWidth=4  IndexOptions=Index vector (dialog)  Indices=4  OutputSizes=1
  Selector1 : Selector  InputPortWidth=4  IndexOptions=Index vector (dialog)  Indices=4  OutputSizes=1
  Yaw cmd : Saturate  UpperLimit=pi  LowerLimit=-pi
  innerLoop_commands : Outport
  wires:
  Bus Selector/1 -> Demux1/1  "<position>"
  Demux1/2 -> Mux/2
  Mux/1 -> Bus Creator/1  "LAP"
  Bus Selector/2 -> Selector1/1, Selector/1  "<params>"
  Selector1/1 -> Yaw cmd/1
  Demux1/1 -> Mux/1
  Hdg. Cmd/1 -> Bus Creator/2  "HeadingCmd"
  Selector/1 -> Hdg. Cmd/1
  Yaw cmd/1 -> Bus Creator/3  "YawCmd"
  Bus Creator/1 -> innerLoop_commands/1
  To/1 -> Bus Selector/1

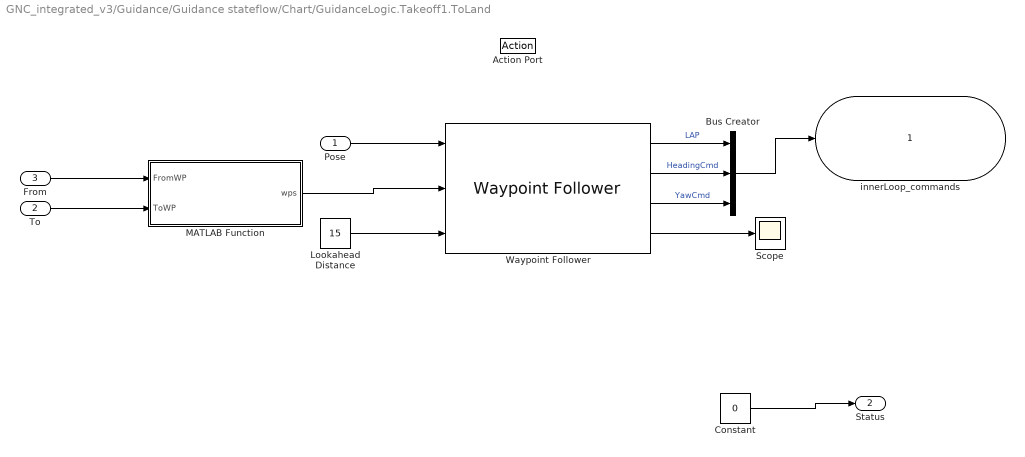
== system GNC_integrated_v3/Guidance/Guidance stateflow/Chart/GuidanceLogic.Takeoff1.ToLand ==
  Pose : Inport
  To : Inport  Port=2
  From : Inport  Port=3
  Action Port : ActionPort
      settings: CopyFcn=Stateflow.SLINSF.SimulinkMan.removeBlockPreDeleteFcn  PreDeleteFcn=Stateflow.SLINSF.SimulinkMan.unsafePredeleteFcn
  Bus Creator : BusCreator  Inputs=3  OutDataTypeStr=Bus: innerLoopCmdsBus  NonVirtualBus=on
  Constant : Constant  Value=0
  Lookahead Distance : Constant  Value=15
  MATLAB Function : MATLAB Function  TreatAsAtomicUnit=on
  Scope : Scope
  Waypoint Follower : uavalgslib/Waypoint Follower  UAVType=multirotor  StartFrom=first  TransitionRadiusSource=internal  TransitionRadius=10  MinLookaheadDistance=0.1  YawInput=off  ShowCrossTrackErrorOutput=off  ShowStatusOutput=off  SimulateUsing=Interpreted execution
  innerLoop_commands : Outport  OutDataTypeStr=Bus: innerLoopCmdsBus
  Status : Outport  Port=2
  wires:
  To/1 -> MATLAB Function/2(ToWP)
  MATLAB Function/1(wps) -> Waypoint Follower/2
  Waypoint Follower/1 -> Bus Creator/1  "LAP"
  Bus Creator/1 -> innerLoop_commands/1
  From/1 -> MATLAB Function/1(FromWP)
  Pose/1 -> Waypoint Follower/1
  Waypoint Follower/2 -> Bus Creator/2  "HeadingCmd"
  Waypoint Follower/4 -> Scope/1
  Lookahead Distance/1 -> Waypoint Follower/3
  Waypoint Follower/3 -> Bus Creator/3  "YawCmd"
  Constant/1 -> Status/1

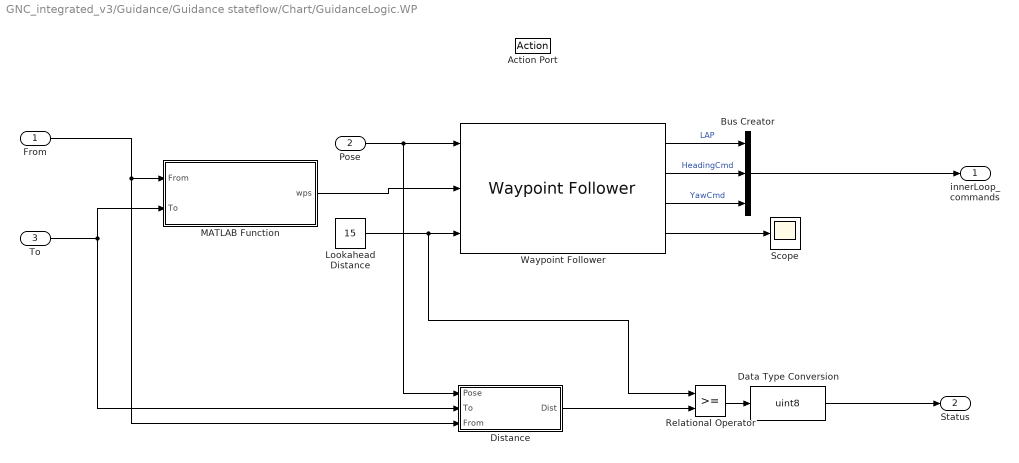
== system GNC_integrated_v3/Guidance/Guidance stateflow/Chart/GuidanceLogic.WP ==
  From : Inport
  Pose : Inport  Port=2
  To : Inport  Port=3
  Action Port : ActionPort
      settings: CopyFcn=Stateflow.SLINSF.SimulinkMan.removeBlockPreDeleteFcn  PreDeleteFcn=Stateflow.SLINSF.SimulinkMan.unsafePredeleteFcn
  Bus Creator : BusCreator  Inputs=3  OutDataTypeStr=Bus: innerLoopCmdsBus  NonVirtualBus=on
  Data Type Conversion : DataTypeConversion  OutDataTypeStr=uint8  SaturateOnIntegerOverflow=off  RndMeth=Floor
  Distance : Subsystem
  Lookahead Distance : Constant  Value=15  OutDataTypeStr=single
  MATLAB Function : MATLAB Function  TreatAsAtomicUnit=on
  Relational Operator : RelationalOperator  OutDataTypeStr=boolean  RndMeth=Simplest  InputSameDT=off
  Scope : Scope
  Waypoint Follower : uavalgslib/Waypoint Follower  UAVType=multirotor  StartFrom=first  TransitionRadiusSource=internal  TransitionRadius=10  MinLookaheadDistance=0.1  YawInput=off  ShowCrossTrackErrorOutput=off  ShowStatusOutput=off  SimulateUsing=Interpreted execution
  innerLoop_commands : Outport  OutDataTypeStr=Bus: innerLoopCmdsBus
  Status : Outport  Port=2
  wires:
  To/1 -> MATLAB Function/2(To), Distance/2(To)
  MATLAB Function/1(wps) -> Waypoint Follower/2
  Waypoint Follower/1 -> Bus Creator/1  "LAP"
  Data Type Conversion/1 -> Status/1
  Bus Creator/1 -> innerLoop_commands/1
  From/1 -> Distance/3(From), MATLAB Function/1(From)
  Pose/1 -> Distance/1(Pose), Waypoint Follower/1
  Waypoint Follower/2 -> Bus Creator/2  "HeadingCmd"
  Waypoint Follower/4 -> Scope/1
  Relational Operator/1 -> Data Type Conversion/1
  Distance/1(Dist) -> Relational Operator/2
  Lookahead Distance/1 -> Relational Operator/1, Waypoint Follower/3
  Waypoint Follower/3 -> Bus Creator/3  "YawCmd"

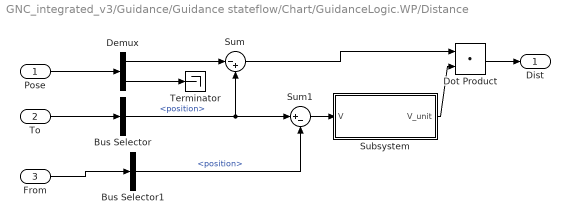
== system GNC_integrated_v3/Guidance/Guidance stateflow/Chart/GuidanceLogic.WP/Distance ==
  Pose : Inport
  To : Inport  Port=2
  From : Inport  Port=3
  Bus Selector : BusSelector  OutputSignals=position
  Bus Selector1 : BusSelector  OutputSignals=position
  Demux : Demux  Outputs=[3 1]
  Dot Product : DotProduct  OutDataTypeStr=Inherit: Inherit via internal rule
  Subsystem : Subsystem
  Sum : Sum  Inputs=|-+
  Sum1 : Sum  Inputs=|+-
  Terminator : Terminator
  Dist : Outport
  wires:
  Pose/1 -> Demux/1
  Demux/1 -> Sum/1
  Demux/2 -> Terminator/1
  To/1 -> Bus Selector/1
  From/1 -> Bus Selector1/1
  Bus Selector1/1 -> Sum1/2  "<position>"
  Bus Selector/1 -> Sum/2, Sum1/1  "<position>"
  Sum/1 -> Dot Product/1
  Dot Product/1 -> Dist/1
  Sum1/1 -> Subsystem/1(V)
  Subsystem/1(V_unit) -> Dot Product/2

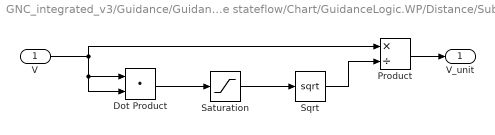
== system GNC_integrated_v3/Guidance/Guidance stateflow/Chart/GuidanceLogic.WP/Distance/Subsystem ==
  V : Inport
  Dot Product : DotProduct  OutDataTypeStr=Inherit: Inherit via internal rule
  Product : Product  Inputs=*/
  Saturation : Saturate
  Sqrt : Sqrt
  V_unit : Outport
  wires:
  Dot Product/1 -> Saturation/1
  Saturation/1 -> Sqrt/1
  V/1 -> Dot Product/1, Dot Product/2, Product/1
  Product/1 -> V_unit/1
  Sqrt/1 -> Product/2

== matlab function GNC_integrated_v3/Guidance/Guidance stateflow/Chart/GuidanceLogic.Takeoff1.ToLand/MATLAB Function ==
  data: FromWP input; wps output; ToWP input
function wps = getLandingWaypoint(FromWP, ToWP)

persistent outWPS

if isempty(outWPS)
    outWPS = single(zeros(2,4));
end

outWPS(1,:) = [FromWP.position' FromWP.params(4)];
outWPS(2,:) = [ToWP.position(1:2)' FromWP.position(3) ToWP.params(4)];

wps = outWPS;

== matlab function GNC_integrated_v3/Guidance/Guidance stateflow/Chart/GuidanceLogic.WP/MATLAB Function ==
  data: From input Bus: UAVPathManagerBus; wps output; To input Bus: UAVPathManagerBus
function wps = getWaypointMission(From, To)

persistent outWPS

if isempty(outWPS)
    outWPS = single(zeros(2,4));
end

outWPS(1,:) = [From.position' From.params(4)];
outWPS(2,:) = [To.position' To.params(4)];

% for ii=1:2
%     outWPS(ii,1:3) = GCSMission(ii).position';
%     outWPS(ii,4) = GCSMission(ii).params(4);
% end

wps = outWPS;

== matlab function GNC_integrated_v3/Navigation/MATLAB Function ==
  data: u input; y output
function y = fcn(u)

y = -[0 -u(3) u(2) ; u(3) 0 -u(1) ; -u(2) u(1) 0 ];

== stateflow chart GNC_integrated_v3/Guidance/Guidance stateflow/Chart ==
  state GuidanceLogic
    state OnGround
    state Takeoff
    state WP
    state Orbit
    state Takeoff1
      state ToLand
      state Descend
      (default) -> ToLand
      ToLand -> Descend
    (default) -> OnGround
    OnGround -> (junction 12) : [startFlight == 1]
    GuidanceLogic -> (junction 12) : [hasChanged(mode)]
    (junction 12) -> Takeoff [order 1] : [mode == 1]
    (junction 12) -> (junction 10) [order 2]
    Takeoff -> WP : [Pose(3) <= To.position(3)]{Status =1;}
    (junction 10) -> WP [order 1] : [mode == 2]
    (junction 10) -> (junction 11) [order 2]
    (junction 11) -> Orbit [order 1] : [mode == 3]
    (junction 11) -> (junction 29) [order 2]
    (junction 29) -> Takeoff1
    Takeoff1 -> GuidanceLogic : [Pose(3)>=-0.1]{Status = 2;}
  (default) -> GuidanceLogic
  data: sf_internal_action_state_placeholder_data local double size=1 =0; sf_internal_action_state_placeholder_data local double size=1 =0; sf_internal_action_state_placeholder_data local double size=1 =0; sf_internal_action_state_placeholder_data local double size=1 =0; sf_internal_action_state_placeholder_data local double size=1 =0; innerLoop_commands output Bus: innerLoopCmdsBus; Status output uint8; mode input uint8; To input Bus: UAVPathManagerBus; From input Bus: UAVPathManagerBus; Pose input; startFlight input
